simulink model "Assignment_3_SL"  (R2016a)
settings: Solver=VariableStepAuto  StartTime=0.0  StopTime=100  RelTol=1e-3
values from neighbouring files (symbols this model uses):
  A = [-1/(R1*A1) 1/(R1*A1); 1/(R1*A2) -(1/A2)*(1/R1 + 1/R2)]    [Eigs.m]
  A1 = 1    [System_parameters.m]
  A2 = 1    [System_parameters.m]
  A_lam = lam    [Eigs.m]
  B = [b1/A1; b2/A2]    [Eigs.m]
  b1 = 0.75    [System_parameters.m]
  b2 = 0.25    [System_parameters.m]
  B_lam = inv(T)*B    [Eigs.m]
  C = eye(2)    [Eigs.m]
  C_lam = C*T    [Eigs.m]
  D = [0; 0]    [Eigs.m]
  R1 = 1    [System_parameters.m]
  R2 = 0.5    [System_parameters.m]
settings Model: Creator=silver_sketcher  LastModifiedBy=silver_sketcher

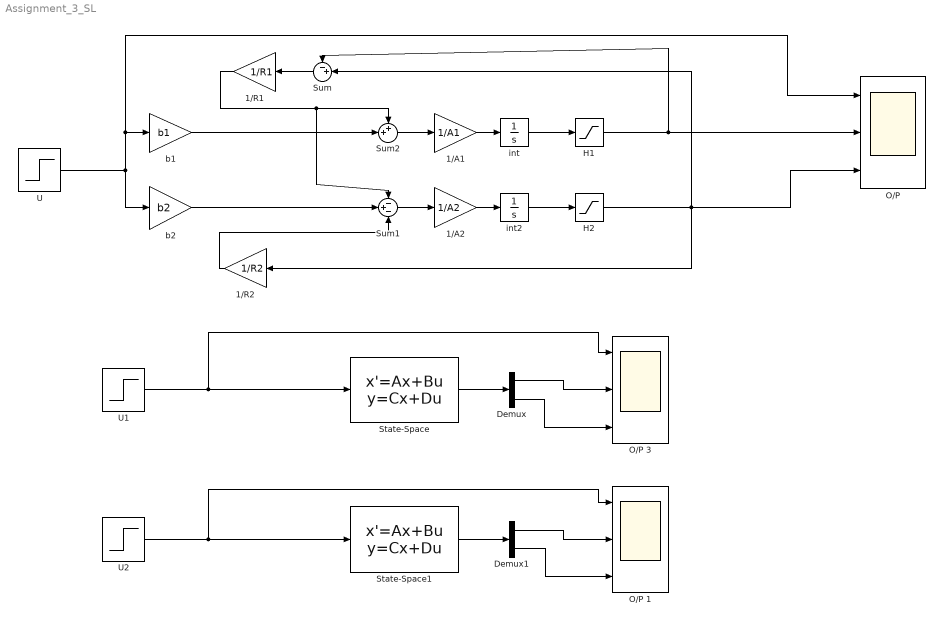
== system Assignment_3_SL ==
  "1/A1 " : Gain  Gain=1/A1
  1/A2 : Gain  Gain=1/A2
  1/R1 : Gain  Gain=1/R1
  "1/R2 " : Gain  Gain=1/R2
  Demux : Demux  Outputs=2
  Demux1 : Demux  Outputs=2
  H1 : Saturate  UpperLimit=inf  LowerLimit=0.0
  H2 : Saturate  UpperLimit=inf  LowerLimit=0.0
  "O/P " : Scope  NumInputPorts=3
  O/P 1 : Scope  NumInputPorts=3
  O/P 3 : Scope  NumInputPorts=3
  State-Space : StateSpace  A=A  B=B  C=C  D=D  X0=0
  State-Space1 : StateSpace  A=A_lam  B=B_lam  C=C_lam  D=D  X0=0
  Sum : Sum  Inputs=-+|
  Sum1 : Sum  Inputs=-+-
  Sum2 : Sum  Inputs=++|
  U : Step  After=u  SampleTime=0
  U1 : Step  After=u  SampleTime=0
  U2 : Step  After=u  SampleTime=0
  b1 : Gain  Gain=b1
  "b2 " : Gain  Gain=b2
  int : Integrator
  int2 : Integrator
  wires:
  U/1 -> "O/P "/1, b1/1, "b2 "/1
  Sum2/1 -> "1/A1 "/1
  Sum1/1 -> 1/A2/1
  "1/A1 "/1 -> int/1
  1/A2/1 -> int2/1
  "b2 "/1 -> Sum1/2
  b1/1 -> Sum2/2
  Sum/1 -> 1/R1/1
  1/R1/1 -> Sum2/1, Sum1/1
  "1/R2 "/1 -> Sum1/3
  State-Space/1 -> Demux/1
  State-Space1/1 -> Demux1/1
  U1/1 -> O/P 3/1, State-Space/1
  Demux/1 -> O/P 3/2
  Demux/2 -> O/P 3/3
  Demux1/1 -> O/P 1/2
  Demux1/2 -> O/P 1/3
  U2/1 -> O/P 1/1, State-Space1/1
  int/1 -> H1/1
  int2/1 -> H2/1
  H1/1 -> "O/P "/2, Sum/1
  H2/1 -> Sum/2, "O/P "/3, "1/R2 "/1
